simulink model "3_ALS_Sterilisation"  (R2023b)
settings: Solver=VariableStepAuto  StartTime=0.0  StopTime=312  RelTol=1e-3
libraries: fl_lib x57, nesl_utility x10, dspstat3 x1
settings Model: Creator=s01mn1  LastModifiedBy=s01mn1

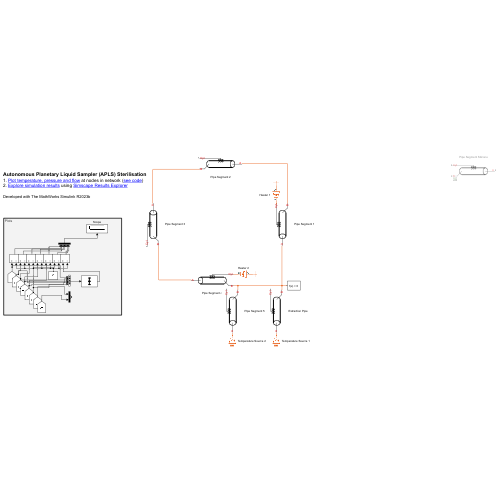
[thumbnail: Simulink's stored preview of the top-level diagram]
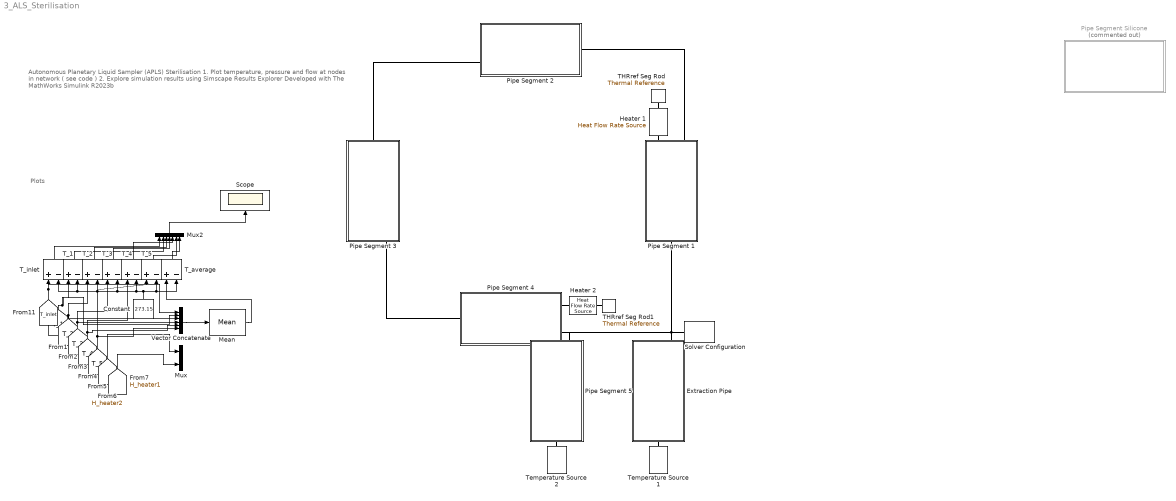
== system 3_ALS_Sterilisation ==
  note: Plots
  note: Autonomous Planetary Liquid Sampler (APLS) Sterilisation
      | 1. Plot temperature, pressure and flow at nodes in network ( see code )
      | 2. Explore simulation results using Simscape Results Explorer
      |
      | Developed with The MathWorks Simulink R2023b
  Constant : Constant  Value=273.15
  Extraction Pipe : Subsystem
      mask Display:
      | % Plot cylinder
      | plot([1,3],[1,1])
      | plot([1,3],[2,2])
      | plot(0.2*cos(0:2*pi/500:2*pi)+1,0.5*sin(0:2*pi/500:2*pi)+1.5)
      | plot(0.2*cos(-pi/2:2*pi/500:pi/2)+3,0.5*sin(-pi/2:2*pi/500:pi/2)+1.5)
      | 
      | % Heat Port
      | plot([1.8 2.2],[2.2 2.2])
      | plot([0.1*cos(-pi/2:0.1:pi/2)+1.8],[0.1*sin(-pi/2:0.1:pi/2)+2.1])
      | plot([0.1*cos(pi/2:0.1:3*pi/2)+1.9],[0.1*sin(pi/2:0.1:3*pi/2)+1.9])
      | plot([0.1*cos(-pi/2:0.1:pi/2)+1.95],[0.1*sin(-pi/2:0.1:pi/2)+2.1])
      | plot([0.1*cos(pi/2:0.1:3*pi/2)+2.05],[0.1*sin(pi/2:0.1:3*pi/2)+1.9])
      | plot([0.1*cos(-pi/2:0.1:pi/2)+2.1],[0.1*sin(-pi/2:0.1:pi/2)+2.1])
      | plot([0.1*cos(pi/2:0.1:3*pi/2)+2.2],[0.1*sin(pi/2:0.1:3*pi/2)+1.9])
      | 
      | % Connecting lines
      | plot([2 3.8],[2.4,2.4])
      | plot([2 2],[2.2 2.4])
      | plot([0.2 1],[1.5 1.5])
      | plot([3.4 3.8],[0.75 0.75])
      | plot([3,3.4],[1.5 0.75])
      | % Scaling
      | color('white')
      | plot(0.2,0)
      | plot(3.8,3.2)
      | 
      | color('red')
      | port_label('Lconn',1,'A')
      | port_label('Rconn',1,'Cyl')
      | port_label('Rconn',2,'B')
  Heater 1 : fl_lib/Thermal/Thermal Sources/Heat Flow Rate Source  heat_flow=60 W
      settings: InternalSimscapePortConfiguration="{\"Bottom\":[],\"Left\":[{\"id\":\"B\",\"label\":\"B\",\"type\":\"foundation.thermal.thermal\"}],\"Right\":[{\"id\":\"A\",\"label\":\"A\",\"type\":\"foundation.thermal.thermal\"}],\"Top\":[]}"
  Heater 2 : fl_lib/Thermal/Thermal Sources/Heat Flow Rate Source  heat_flow=60 W
      settings: InternalSimscapePortConfiguration="{\"Bottom\":[],\"Left\":[{\"id\":\"B\",\"label\":\"B\",\"type\":\"foundation.thermal.thermal\"}],\"Right\":[{\"id\":\"A\",\"label\":\"A\",\"type\":\"foundation.thermal.thermal\"}],\"Top\":[]}"
  Mean : dspstat3/Mean  run=off  InputProcessing=Columns as channels (frame based)  reset_popup=None  directionMode=Each column  dimension=1  roiEnable=off  roiType=Rectangles  roiPortion=Entire ROI  roiOutput=Individual statistics for each ROI  roiFlag=off  roundingMode=Floor  overflowMode=off  outputDataTypeStr=Inherit: Same as accumulator  outputMin=[]  outputMax=[]  outputLastDataTypeStr=Inherit: Same as accumulator
  Mux : Mux  Inputs=2
  Mux2 : Mux  Inputs=7
  Pipe Segment 1 : Subsystem
      mask Display:
      | % Plot cylinder
      | plot([1,3],[1,1])
      | plot([1,3],[2,2])
      | plot(0.2*cos(0:2*pi/500:2*pi)+1,0.5*sin(0:2*pi/500:2*pi)+1.5)
      | plot(0.2*cos(-pi/2:2*pi/500:pi/2)+3,0.5*sin(-pi/2:2*pi/500:pi/2)+1.5)
      | 
      | % Heat Port
      | plot([1.8 2.2],[2.2 2.2])
      | plot([0.1*cos(-pi/2:0.1:pi/2)+1.8],[0.1*sin(-pi/2:0.1:pi/2)+2.1])
      | plot([0.1*cos(pi/2:0.1:3*pi/2)+1.9],[0.1*sin(pi/2:0.1:3*pi/2)+1.9])
      | plot([0.1*cos(-pi/2:0.1:pi/2)+1.95],[0.1*sin(-pi/2:0.1:pi/2)+2.1])
      | plot([0.1*cos(pi/2:0.1:3*pi/2)+2.05],[0.1*sin(pi/2:0.1:3*pi/2)+1.9])
      | plot([0.1*cos(-pi/2:0.1:pi/2)+2.1],[0.1*sin(-pi/2:0.1:pi/2)+2.1])
      | plot([0.1*cos(pi/2:0.1:3*pi/2)+2.2],[0.1*sin(pi/2:0.1:3*pi/2)+1.9])
      | 
      | % Connecting lines
      | plot([2 3.8],[2.4,2.4])
      | plot([2 2],[2.2 2.4])
      | plot([0.2 1],[1.5 1.5])
      | plot([3.4 3.8],[0.75 0.75])
      | plot([3,3.4],[1.5 0.75])
      | % Scaling
      | color('white')
      | plot(0.2,0)
      | plot(3.8,3.2)
      | 
      | color('red')
      | port_label('Lconn',1,'A')
      | port_label('Rconn',1,'Cyl')
      | port_label('Rconn',2,'B')
  Pipe Segment 2 : Subsystem
      mask Display:
      | % Plot cylinder
      | plot([1,3],[1,1])
      | plot([1,3],[2,2])
      | plot(0.2*cos(0:2*pi/500:2*pi)+1,0.5*sin(0:2*pi/500:2*pi)+1.5)
      | plot(0.2*cos(-pi/2:2*pi/500:pi/2)+3,0.5*sin(-pi/2:2*pi/500:pi/2)+1.5)
      | 
      | % Heat Port
      | plot([1.8 2.2],[2.2 2.2])
      | plot([0.1*cos(-pi/2:0.1:pi/2)+1.8],[0.1*sin(-pi/2:0.1:pi/2)+2.1])
      | plot([0.1*cos(pi/2:0.1:3*pi/2)+1.9],[0.1*sin(pi/2:0.1:3*pi/2)+1.9])
      | plot([0.1*cos(-pi/2:0.1:pi/2)+1.95],[0.1*sin(-pi/2:0.1:pi/2)+2.1])
      | plot([0.1*cos(pi/2:0.1:3*pi/2)+2.05],[0.1*sin(pi/2:0.1:3*pi/2)+1.9])
      | plot([0.1*cos(-pi/2:0.1:pi/2)+2.1],[0.1*sin(-pi/2:0.1:pi/2)+2.1])
      | plot([0.1*cos(pi/2:0.1:3*pi/2)+2.2],[0.1*sin(pi/2:0.1:3*pi/2)+1.9])
      | 
      | % Connecting lines
      | plot([2 3.8],[2.4,2.4])
      | plot([2 2],[2.2 2.4])
      | plot([0.2 1],[1.5 1.5])
      | plot([3.4 3.8],[0.75 0.75])
      | plot([3,3.4],[1.5 0.75])
      | % Scaling
      | color('white')
      | plot(0.2,0)
      | plot(3.8,3.2)
      | 
      | color('red')
      | port_label('Lconn',1,'A')
      | port_label('Rconn',1,'Cyl')
      | port_label('Rconn',2,'B')
  Pipe Segment 3 : Subsystem
      mask Display:
      | % Plot cylinder
      | plot([1,3],[1,1])
      | plot([1,3],[2,2])
      | plot(0.2*cos(0:2*pi/500:2*pi)+1,0.5*sin(0:2*pi/500:2*pi)+1.5)
      | plot(0.2*cos(-pi/2:2*pi/500:pi/2)+3,0.5*sin(-pi/2:2*pi/500:pi/2)+1.5)
      | 
      | % Heat Port
      | plot([1.8 2.2],[2.2 2.2])
      | plot([0.1*cos(-pi/2:0.1:pi/2)+1.8],[0.1*sin(-pi/2:0.1:pi/2)+2.1])
      | plot([0.1*cos(pi/2:0.1:3*pi/2)+1.9],[0.1*sin(pi/2:0.1:3*pi/2)+1.9])
      | plot([0.1*cos(-pi/2:0.1:pi/2)+1.95],[0.1*sin(-pi/2:0.1:pi/2)+2.1])
      | plot([0.1*cos(pi/2:0.1:3*pi/2)+2.05],[0.1*sin(pi/2:0.1:3*pi/2)+1.9])
      | plot([0.1*cos(-pi/2:0.1:pi/2)+2.1],[0.1*sin(-pi/2:0.1:pi/2)+2.1])
      | plot([0.1*cos(pi/2:0.1:3*pi/2)+2.2],[0.1*sin(pi/2:0.1:3*pi/2)+1.9])
      | 
      | % Connecting lines
      | plot([2 3.8],[2.4,2.4])
      | plot([2 2],[2.2 2.4])
      | plot([0.2 1],[1.5 1.5])
      | plot([3.4 3.8],[0.75 0.75])
      | plot([3,3.4],[1.5 0.75])
      | % Scaling
      | color('white')
      | plot(0.2,0)
      | plot(3.8,3.2)
      | 
      | color('red')
      | port_label('Lconn',1,'A')
      | port_label('Rconn',1,'Cyl')
      | port_label('Rconn',2,'B')
  Pipe Segment 4 : Subsystem
      mask Display:
      | % Plot cylinder
      | plot([1,3],[1,1])
      | plot([1,3],[2,2])
      | plot(0.2*cos(0:2*pi/500:2*pi)+1,0.5*sin(0:2*pi/500:2*pi)+1.5)
      | plot(0.2*cos(-pi/2:2*pi/500:pi/2)+3,0.5*sin(-pi/2:2*pi/500:pi/2)+1.5)
      | 
      | % Heat Port
      | plot([1.8 2.2],[2.2 2.2])
      | plot([0.1*cos(-pi/2:0.1:pi/2)+1.8],[0.1*sin(-pi/2:0.1:pi/2)+2.1])
      | plot([0.1*cos(pi/2:0.1:3*pi/2)+1.9],[0.1*sin(pi/2:0.1:3*pi/2)+1.9])
      | plot([0.1*cos(-pi/2:0.1:pi/2)+1.95],[0.1*sin(-pi/2:0.1:pi/2)+2.1])
      | plot([0.1*cos(pi/2:0.1:3*pi/2)+2.05],[0.1*sin(pi/2:0.1:3*pi/2)+1.9])
      | plot([0.1*cos(-pi/2:0.1:pi/2)+2.1],[0.1*sin(-pi/2:0.1:pi/2)+2.1])
      | plot([0.1*cos(pi/2:0.1:3*pi/2)+2.2],[0.1*sin(pi/2:0.1:3*pi/2)+1.9])
      | 
      | % Connecting lines
      | plot([2 3.8],[2.4,2.4])
      | plot([2 2],[2.2 2.4])
      | plot([0.2 1],[1.5 1.5])
      | plot([3.4 3.8],[0.75 0.75])
      | plot([3,3.4],[1.5 0.75])
      | % Scaling
      | color('white')
      | plot(0.2,0)
      | plot(3.8,3.2)
      | 
      | color('red')
      | port_label('Lconn',1,'A')
      | port_label('Rconn',1,'Cyl')
      | port_label('Rconn',2,'B')
  Pipe Segment 5 : Subsystem
      mask Display:
      | % Plot cylinder
      | plot([1,3],[1,1])
      | plot([1,3],[2,2])
      | plot(0.2*cos(0:2*pi/500:2*pi)+1,0.5*sin(0:2*pi/500:2*pi)+1.5)
      | plot(0.2*cos(-pi/2:2*pi/500:pi/2)+3,0.5*sin(-pi/2:2*pi/500:pi/2)+1.5)
      | 
      | % Heat Port
      | plot([1.8 2.2],[2.2 2.2])
      | plot([0.1*cos(-pi/2:0.1:pi/2)+1.8],[0.1*sin(-pi/2:0.1:pi/2)+2.1])
      | plot([0.1*cos(pi/2:0.1:3*pi/2)+1.9],[0.1*sin(pi/2:0.1:3*pi/2)+1.9])
      | plot([0.1*cos(-pi/2:0.1:pi/2)+1.95],[0.1*sin(-pi/2:0.1:pi/2)+2.1])
      | plot([0.1*cos(pi/2:0.1:3*pi/2)+2.05],[0.1*sin(pi/2:0.1:3*pi/2)+1.9])
      | plot([0.1*cos(-pi/2:0.1:pi/2)+2.1],[0.1*sin(-pi/2:0.1:pi/2)+2.1])
      | plot([0.1*cos(pi/2:0.1:3*pi/2)+2.2],[0.1*sin(pi/2:0.1:3*pi/2)+1.9])
      | 
      | % Connecting lines
      | plot([2 3.8],[2.4,2.4])
      | plot([2 2],[2.2 2.4])
      | plot([0.2 1],[1.5 1.5])
      | plot([3.4 3.8],[0.75 0.75])
      | plot([3,3.4],[1.5 0.75])
      | % Scaling
      | color('white')
      | plot(0.2,0)
      | plot(3.8,3.2)
      | 
      | color('red')
      | port_label('Lconn',1,'A')
      | port_label('Rconn',1,'Cyl')
      | port_label('Rconn',2,'B')
  Pipe Segment Silicone : Subsystem  Commented=on
      mask Display:
      | % Plot cylinder
      | plot([1,3],[1,1])
      | plot([1,3],[2,2])
      | plot(0.2*cos(0:2*pi/500:2*pi)+1,0.5*sin(0:2*pi/500:2*pi)+1.5)
      | plot(0.2*cos(-pi/2:2*pi/500:pi/2)+3,0.5*sin(-pi/2:2*pi/500:pi/2)+1.5)
      | 
      | % Heat Port
      | plot([1.8 2.2],[2.2 2.2])
      | plot([0.1*cos(-pi/2:0.1:pi/2)+1.8],[0.1*sin(-pi/2:0.1:pi/2)+2.1])
      | plot([0.1*cos(pi/2:0.1:3*pi/2)+1.9],[0.1*sin(pi/2:0.1:3*pi/2)+1.9])
      | plot([0.1*cos(-pi/2:0.1:pi/2)+1.95],[0.1*sin(-pi/2:0.1:pi/2)+2.1])
      | plot([0.1*cos(pi/2:0.1:3*pi/2)+2.05],[0.1*sin(pi/2:0.1:3*pi/2)+1.9])
      | plot([0.1*cos(-pi/2:0.1:pi/2)+2.1],[0.1*sin(-pi/2:0.1:pi/2)+2.1])
      | plot([0.1*cos(pi/2:0.1:3*pi/2)+2.2],[0.1*sin(pi/2:0.1:3*pi/2)+1.9])
      | 
      | % Connecting lines
      | plot([2 3.8],[2.4,2.4])
      | plot([2 2],[2.2 2.4])
      | plot([0.2 1],[1.5 1.5])
      | plot([3.4 3.8],[0.75 0.75])
      | plot([3,3.4],[1.5 0.75])
      | % Scaling
      | color('white')
      | plot(0.2,0)
      | plot(3.8,3.2)
      | 
      | color('red')
      | port_label('Lconn',1,'A')
      | port_label('Rconn',1,'Cyl')
      | port_label('Rconn',2,'B')
  Scope : Scope
  Solver Configuration : nesl_utility/Solver Configuration  PhysicalDomain=network_engine_domain  SubClassName=solver  LeftPortType=input  RightPortType=generic  Tones=[]  Harmonics=[]  SimulateNoise=off  Profile=off  UseLocalSampling=off  EnableSwitchedLinearOptims=on  FrequencyDomain=off  UseCCode=off  RelTol=0.001  AbsTol=0.001  MinStep=1e-09  ToWorkspace=off  RevertToSquareIcSolve=off  NumHomotopyIterations=100  PhasorMode=off  PhasorModeNumHarmonics=1  ConsistencySolver=NEWTON_XTOL_AFTER_FTOL  IndexReductionMethod=DerivativeReplacement  DoDC=off  ResidualTolerance=1e-09  ConsistencyTolSource=GLOBAL  ConsistencyAbsTol=0.001  ConsistencyRelTol=0.001  ConsistencyTolFactor=0.001  UseLocalSolver=off  LocalSolverChoice=NE_BACKWARD_EULER_ADVANCER  ResolveIndetEquations=on  FunctionEvalNumThread=1  LocalSolverSampleTime=0.001  DoFixedCost=off  MaxNonlinIter=3  MaxModeIter=2  ComputeImpulses=off  ImpulseIterations=2  LinearAlgebra=auto  LinearAlgebraNumThread=0  EquationFormulation=NE_TIME_EF  DelaysMemoryBudget=1024  AutomaticFiltering=on  FilteringTimeConstant=0.001  PartitionStorageMethod=AS_NEEDED  PartitionMemoryBudget=1024  PartitionMethod=ROBUST  MultibodyUseLocalSolver=off  MultibodyLocalSolverChoice=ODE1  MultibodyLocalSolverSampleTime=0.001
  THRref Seg Rod : fl_lib/Thermal/Thermal Elements/Thermal Reference
  THRref Seg Rod1 : fl_lib/Thermal/Thermal Elements/Thermal Reference
  T_{1..5} (5 alike) : Sum  Inputs=+-
  T_average : Sum  Inputs=+-
  T_inlet : Sum  Inputs=+-
  Temperature Source 1 : fl_lib/Thermal/Thermal Sources/Temperature Source  temperature=30 degC
  Temperature Source 2 : fl_lib/Thermal/Thermal Sources/Temperature Source  temperature=30 degC
  Vector Concatenate : Concatenate  NumInputs=6
  wires:
  Constant/1 -> T_inlet/2, T_1/2, T_2/2, T_3/2, T_4/2, T_average/2, T_5/2
  Mux2/1 -> Scope/1
  [T_inlet] -> Vector Concatenate/1, T_inlet/1
  [T_1] -> Vector Concatenate/2, T_1/1
  [T_2] -> T_2/1, Vector Concatenate/3
  [T_3] -> T_3/1, Vector Concatenate/4
  T_inlet/1 -> Mux2/1
  T_1/1 -> Mux2/2
  T_2/1 -> Mux2/3
  T_3/1 -> Mux2/4
  [T_4] -> Vector Concatenate/5, T_4/1
  T_4/1 -> Mux2/5
  [T_5] -> Vector Concatenate/6, T_5/1
  T_5/1 -> Mux2/6
  [H_heater2] -> Mux/1
  [H_heater1] -> Mux/2
  T_average/1 -> Mux2/7
  Vector Concatenate/1 -> Mean/1
  Mean/1 -> T_average/1
  connections:
  Heater 1/LConn1 -- Pipe Segment 1/RConn1
  THRref Seg Rod/LConn1 -- Heater 1/RConn1
  Solver Configuration/RConn1 -- Pipe Segment 4/RConn2 -- Pipe Segment 5/RConn2 -- Extraction Pipe/RConn2 -- Pipe Segment 1/LConn1
  Pipe Segment 4/LConn1 -- Pipe Segment 3/RConn2
  THRref Seg Rod1/LConn1 -- Heater 2/RConn1
  Heater 2/LConn1 -- Pipe Segment 4/RConn1
  Pipe Segment 3/LConn1 -- Pipe Segment 2/RConn2
  Pipe Segment 2/LConn1 -- Pipe Segment 1/RConn2
  Temperature Source 1/LConn1 -- Extraction Pipe/LConn1
  Temperature Source 2/LConn1 -- Pipe Segment 5/LConn1

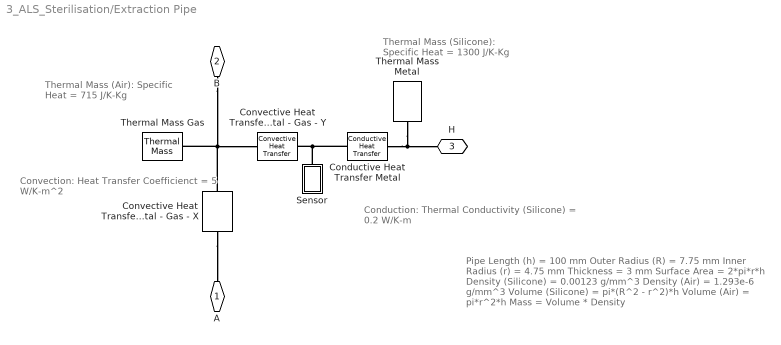
== system 3_ALS_Sterilisation/Extraction Pipe ==
  note: Thermal Mass (Silicone):
      | Specific Heat = 1300 J/K-Kg
  note: Thermal Mass  (Air):
      | Specific Heat = 715 J/K-Kg
  note: Pipe Length (h) = 100 mm
      | Outer Radius (R) = 7.75 mm
      | Inner Radius (r) = 4.75 mm
      | Thickness = 3 mm
      | Surface Area = 2*pi*r*h
      | Density (Silicone) = 0.00123 g/mm^3
      | Density (Air) = 1.293e-6 g/mm^3
      | Volume (Silicone) = pi*(R^2 - r^2)*h
      | Volume (Air) = pi*r^2*h
      | Mass = Volume * Density
  note: Conduction:
      | Thermal Conductivity (Silicone) = 0.2 W/K-m
  note: Convection:
      | Heat Transfer Coefficienct = 5 W/K-m^2
  Conductive Heat Transfer Metal : fl_lib/Thermal/Thermal Elements/Conductive Heat Transfer  thermal_type=foundation.enum.ConstantVariableTabulated.Constant  wall_geometry=foundation.enum.ConductionWallGeometry.Planar  area=7461.282 mm^2  thickness=3 mm  d_in=0.05 m  d_out=0.1 m  L=1 m  th_cond_min=10 W/(K*m)  th_cond=0.2 W/(K*m)  th_cond_TLU=[413, 401, 392, 383, 371, 357, 342] W/(K*m)  temp_TLU=[200, 273, 400, 600, 800, 1000, 1200] K  T_specify=on  T_priority=None  T=30 degC  T_nominal_specify=off  T_nominal_unit=K  T_nominal_value=1  Q_specify=off  Q_priority=None  Q=0 W  Q_nominal_specify=off  Q_nominal_unit=W  Q_nominal_value=1
  Convective Heat Transfer Metal - Gas - X : fl_lib/Thermal/Thermal Elements/Convective Heat Transfer  thermal_type=foundation.enum.constant_variable.constant  area=7461.282 mm^2  heat_tr_coeff=5 W/(K*m^2)  min_heat_tr_coeff=1e-3 W/(K*m^2)  T_specify=on  T_priority=None  T=30 degC  T_nominal_specify=off  T_nominal_unit=K  T_nominal_value=1  Q_specify=off  Q_priority=None  Q=0 W  Q_nominal_specify=off  Q_nominal_unit=W  Q_nominal_value=1
  Convective Heat Transfer Metal - Gas - Y : fl_lib/Thermal/Thermal Elements/Convective Heat Transfer  thermal_type=foundation.enum.constant_variable.constant  area=7461.282 mm^2  heat_tr_coeff=5 W/(K*m^2)  min_heat_tr_coeff=1e-3 W/(K*m^2)  T_specify=on  T_priority=None  T=30 degC  T_nominal_specify=off  T_nominal_unit=K  T_nominal_value=1  Q_specify=off  Q_priority=None  Q=0 W  Q_nominal_specify=off  Q_nominal_unit=W  Q_nominal_value=1
  Sensor : Subsystem
  Thermal Mass Gas : fl_lib/Thermal/Thermal Elements/Thermal Mass  mass_type=foundation.enum.constant_variable.constant  mass=0.0229 g  sp_heat=715 J/(K*kg)  mass_min=1e-6 kg  num_ports=foundation.enum.numPorts2.one  m_specify=off  m_priority=High  m=1 kg  m_nominal_specify=off  m_nominal_unit=kg  m_nominal_value=1  T_specify=on  T_priority=High  T=30 degC  T_nominal_specify=off  T_nominal_unit=K  T_nominal_value=1  Q_specify=off  Q_priority=None  Q=0 W  Q_nominal_specify=off  Q_nominal_unit=W  Q_nominal_value=1
  Thermal Mass Metal : fl_lib/Thermal/Thermal Elements/Thermal Mass  mass_type=foundation.enum.constant_variable.constant  mass=36.2265 g  sp_heat=1300 J/(K*kg)  mass_min=1e-6 kg  num_ports=foundation.enum.numPorts2.one  m_specify=off  m_priority=High  m=1 kg  m_nominal_specify=off  m_nominal_unit=kg  m_nominal_value=1  T_specify=on  T_priority=High  T=30 degC  T_nominal_specify=off  T_nominal_unit=K  T_nominal_value=1  Q_specify=off  Q_priority=None  Q=0 W  Q_nominal_specify=off  Q_nominal_unit=W  Q_nominal_value=1
  A : PMIOPort  Side=Left
  B : PMIOPort  Port=2  Side=Right
  H : PMIOPort  Port=3  Side=Right
  connections:
  Thermal Mass Metal/LConn1 -- H/RConn1 -- Conductive Heat Transfer Metal/LConn1
  Convective Heat Transfer Metal - Gas - X/RConn1 -- Thermal Mass Gas/LConn1 -- Convective Heat Transfer Metal - Gas - Y/RConn1 -- B/RConn1
  Sensor/LConn1 -- Convective Heat Transfer Metal - Gas - Y/LConn1 -- Conductive Heat Transfer Metal/RConn1
  Convective Heat Transfer Metal - Gas - X/LConn1 -- A/RConn1

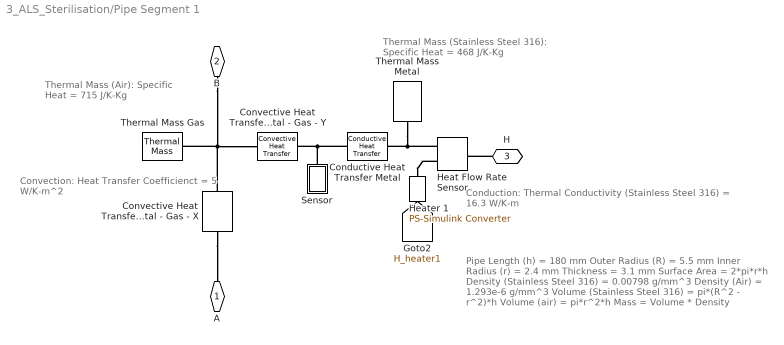
== system 3_ALS_Sterilisation/Pipe Segment 1 ==
  note: Pipe Length (h) = 180 mm
      | Outer Radius (R) = 5.5 mm
      | Inner Radius (r) = 2.4 mm
      | Thickness = 3.1 mm
      | Surface Area = 2*pi*r*h
      | Density (Stainless Steel 316) = 0.00798 g/mm^3
      | Density (Air) = 1.293e-6 g/mm^3
      | Volume (Stainless Steel 316) = pi*(R^2 - r^2)*h
      | Volume (air) = pi*r^2*h
      | Mass = Volume * Density
  note: Thermal Mass (Stainless Steel 316):
      | Specific Heat = 468 J/K-Kg
  note: Conduction:
      | Thermal Conductivity (Stainless Steel 316) = 16.3 W/K-m
  note: Convection:
      | Heat Transfer Coefficienct = 5 W/K-m^2
  note: Thermal Mass  (Air):
      | Specific Heat = 715 J/K-Kg
  Conductive Heat Transfer Metal : fl_lib/Thermal/Thermal Elements/Conductive Heat Transfer  thermal_type=foundation.enum.ConstantVariableTabulated.Constant  wall_geometry=foundation.enum.ConductionWallGeometry.Planar  area=2714.336 mm^2  thickness=3.1 mm  d_in=0.05 m  d_out=0.1 m  L=1 m  th_cond_min=10 W/(K*m)  th_cond=16.3 W/(K*m)  th_cond_TLU=[413, 401, 392, 383, 371, 357, 342] W/(K*m)  temp_TLU=[200, 273, 400, 600, 800, 1000, 1200] K  T_specify=on  T_priority=None  T=30 degC  T_nominal_specify=off  T_nominal_unit=K  T_nominal_value=1  Q_specify=off  Q_priority=None  Q=0 W  Q_nominal_specify=off  Q_nominal_unit=W  Q_nominal_value=1
  Convective Heat Transfer Metal - Gas - X : fl_lib/Thermal/Thermal Elements/Convective Heat Transfer  thermal_type=foundation.enum.constant_variable.constant  area=2714.336 mm^2  heat_tr_coeff=5 W/(K*m^2)  min_heat_tr_coeff=1e-3 W/(K*m^2)  T_specify=on  T_priority=None  T=30 degC  T_nominal_specify=off  T_nominal_unit=K  T_nominal_value=1  Q_specify=off  Q_priority=None  Q=0 W  Q_nominal_specify=off  Q_nominal_unit=W  Q_nominal_value=1
  Convective Heat Transfer Metal - Gas - Y : fl_lib/Thermal/Thermal Elements/Convective Heat Transfer  thermal_type=foundation.enum.constant_variable.constant  area=2714.336 mm^2  heat_tr_coeff=5 W/(K*m^2)  min_heat_tr_coeff=1e-3 W/(K*m^2)  T_specify=on  T_priority=None  T=30 degC  T_nominal_specify=off  T_nominal_unit=K  T_nominal_value=1  Q_specify=off  Q_priority=None  Q=0 W  Q_nominal_specify=off  Q_nominal_unit=W  Q_nominal_value=1
  Heat Flow Rate Sensor : fl_lib/Thermal/Thermal Sensors/Heat Flow Rate Sensor
  Heater 1 : nesl_utility/PS-Simulink Converter  PhysicalDomain=network_engine_domain  SubClassName=ps_output  LeftPortType=input  RightPortType=output  PseudoPeriodic=off  Frequencies=[]  VectorFormat=inherit  Unit=inherit  AffineConversion=off
  Sensor : Subsystem
  Thermal Mass Gas : fl_lib/Thermal/Thermal Elements/Thermal Mass  mass_type=foundation.enum.constant_variable.constant  mass=0.0042 g  sp_heat=715 J/(K*kg)  mass_min=1e-6 kg  num_ports=foundation.enum.numPorts2.one  m_specify=off  m_priority=High  m=1 kg  m_nominal_specify=off  m_nominal_unit=kg  m_nominal_value=1  T_specify=on  T_priority=High  T=30 degC  T_nominal_specify=off  T_nominal_unit=K  T_nominal_value=1  Q_specify=off  Q_priority=None  Q=0 W  Q_nominal_specify=off  Q_nominal_unit=W  Q_nominal_value=1
  Thermal Mass Metal : fl_lib/Thermal/Thermal Elements/Thermal Mass  mass_type=foundation.enum.constant_variable.constant  mass=110.5132 g  sp_heat=468 J/(K*kg)  mass_min=1e-6 kg  num_ports=foundation.enum.numPorts2.one  m_specify=off  m_priority=High  m=1 kg  m_nominal_specify=off  m_nominal_unit=kg  m_nominal_value=1  T_specify=on  T_priority=High  T=30 degC  T_nominal_specify=off  T_nominal_unit=K  T_nominal_value=1  Q_specify=off  Q_priority=None  Q=0 W  Q_nominal_specify=off  Q_nominal_unit=W  Q_nominal_value=1
  A : PMIOPort  Side=Left
  B : PMIOPort  Port=2  Side=Right
  H : PMIOPort  Port=3  Side=Right
  tag scope: H_heater1=global
  wires:
  Heater 1/1 -> [H_heater1]
  connections:
  Conductive Heat Transfer Metal/RConn1 -- Convective Heat Transfer Metal - Gas - Y/LConn1 -- Sensor/LConn1
  Thermal Mass Metal/LConn1 -- Heat Flow Rate Sensor/RConn2 -- Conductive Heat Transfer Metal/LConn1
  Convective Heat Transfer Metal - Gas - X/LConn1 -- A/RConn1
  Convective Heat Transfer Metal - Gas - X/RConn1 -- B/RConn1 -- Thermal Mass Gas/LConn1 -- Convective Heat Transfer Metal - Gas - Y/RConn1
  Heat Flow Rate Sensor/RConn1 -- Heater 1/LConn1
  H/RConn1 -- Heat Flow Rate Sensor/LConn1

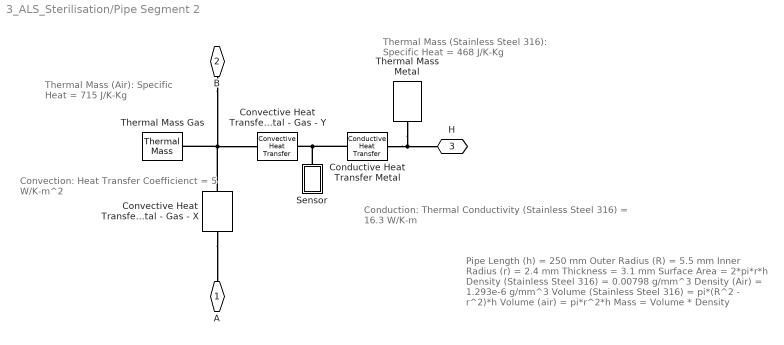
== system 3_ALS_Sterilisation/Pipe Segment 2 ==
  note: Convection:
      | Heat Transfer Coefficienct = 5 W/K-m^2
  note: Thermal Mass (Stainless Steel 316):
      | Specific Heat = 468 J/K-Kg
  note: Conduction:
      | Thermal Conductivity (Stainless Steel 316) = 16.3 W/K-m
  note: Thermal Mass  (Air):
      | Specific Heat = 715 J/K-Kg
  note: Pipe Length (h) = 250 mm
      | Outer Radius (R) = 5.5 mm
      | Inner Radius (r) = 2.4 mm
      | Thickness = 3.1 mm
      | Surface Area = 2*pi*r*h
      | Density (Stainless Steel 316) = 0.00798 g/mm^3
      | Density (Air) = 1.293e-6 g/mm^3
      | Volume (Stainless Steel 316) = pi*(R^2 - r^2)*h
      | Volume (air) = pi*r^2*h
      | Mass = Volume * Density
  Conductive Heat Transfer Metal : fl_lib/Thermal/Thermal Elements/Conductive Heat Transfer  thermal_type=foundation.enum.ConstantVariableTabulated.Constant  wall_geometry=foundation.enum.ConductionWallGeometry.Planar  area=3769.911 mm^2  thickness=3.1 mm  d_in=0.05 m  d_out=0.1 m  L=1 m  th_cond_min=10 W/(K*m)  th_cond=16.3 W/(K*m)  th_cond_TLU=[413, 401, 392, 383, 371, 357, 342] W/(K*m)  temp_TLU=[200, 273, 400, 600, 800, 1000, 1200] K  T_specify=on  T_priority=None  T=30 degC  T_nominal_specify=off  T_nominal_unit=K  T_nominal_value=1  Q_specify=off  Q_priority=None  Q=0 W  Q_nominal_specify=off  Q_nominal_unit=W  Q_nominal_value=1
  Convective Heat Transfer Metal - Gas - X : fl_lib/Thermal/Thermal Elements/Convective Heat Transfer  thermal_type=foundation.enum.constant_variable.constant  area=3769.911 mm^2  heat_tr_coeff=5 W/(K*m^2)  min_heat_tr_coeff=1e-3 W/(K*m^2)  T_specify=on  T_priority=None  T=30 degC  T_nominal_specify=off  T_nominal_unit=K  T_nominal_value=1  Q_specify=off  Q_priority=None  Q=0 W  Q_nominal_specify=off  Q_nominal_unit=W  Q_nominal_value=1
  Convective Heat Transfer Metal - Gas - Y : fl_lib/Thermal/Thermal Elements/Convective Heat Transfer  thermal_type=foundation.enum.constant_variable.constant  area=3769.911 mm^2  heat_tr_coeff=5 W/(K*m^2)  min_heat_tr_coeff=1e-3 W/(K*m^2)  T_specify=on  T_priority=None  T=30 degC  T_nominal_specify=off  T_nominal_unit=K  T_nominal_value=1  Q_specify=off  Q_priority=None  Q=0 W  Q_nominal_specify=off  Q_nominal_unit=W  Q_nominal_value=1
  Sensor : Subsystem
  Thermal Mass Gas : fl_lib/Thermal/Thermal Elements/Thermal Mass  mass_type=foundation.enum.constant_variable.constant  mass=0.0058 g  sp_heat=715 J/(K*kg)  mass_min=1e-6 kg  num_ports=foundation.enum.numPorts2.one  m_specify=off  m_priority=High  m=1 kg  m_nominal_specify=off  m_nominal_unit=kg  m_nominal_value=1  T_specify=on  T_priority=High  T=30 degC  T_nominal_specify=off  T_nominal_unit=K  T_nominal_value=1  Q_specify=off  Q_priority=None  Q=0 W  Q_nominal_specify=off  Q_nominal_unit=W  Q_nominal_value=1
  Thermal Mass Metal : fl_lib/Thermal/Thermal Elements/Thermal Mass  mass_type=foundation.enum.constant_variable.constant  mass=153.4905 g  sp_heat=468 J/(K*kg)  mass_min=1e-6 kg  num_ports=foundation.enum.numPorts2.one  m_specify=off  m_priority=High  m=1 kg  m_nominal_specify=off  m_nominal_unit=kg  m_nominal_value=1  T_specify=on  T_priority=High  T=30 degC  T_nominal_specify=off  T_nominal_unit=K  T_nominal_value=1  Q_specify=off  Q_priority=None  Q=0 W  Q_nominal_specify=off  Q_nominal_unit=W  Q_nominal_value=1
  A : PMIOPort  Side=Left
  B : PMIOPort  Port=2  Side=Right
  H : PMIOPort  Port=3  Side=Right
  connections:
  Convective Heat Transfer Metal - Gas - X/RConn1 -- Thermal Mass Gas/LConn1 -- Convective Heat Transfer Metal - Gas - Y/RConn1 -- B/RConn1
  Sensor/LConn1 -- Convective Heat Transfer Metal - Gas - Y/LConn1 -- Conductive Heat Transfer Metal/RConn1
  Thermal Mass Metal/LConn1 -- H/RConn1 -- Conductive Heat Transfer Metal/LConn1
  Convective Heat Transfer Metal - Gas - X/LConn1 -- A/RConn1

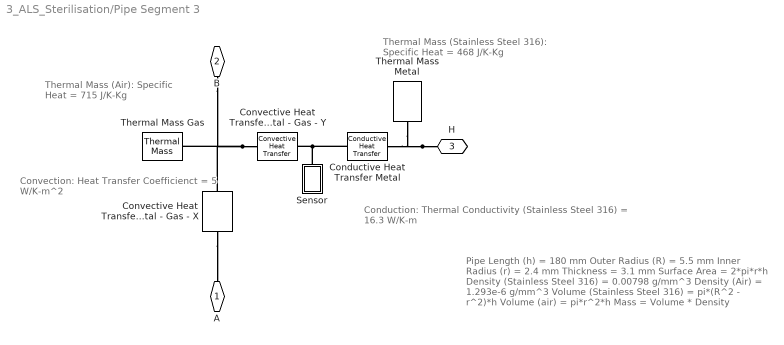
== system 3_ALS_Sterilisation/Pipe Segment 3 ==
  note: Thermal Mass (Stainless Steel 316):
      | Specific Heat = 468 J/K-Kg
  note: Thermal Mass  (Air):
      | Specific Heat = 715 J/K-Kg
  note: Pipe Length (h) = 180 mm
      | Outer Radius (R) = 5.5 mm
      | Inner Radius (r) = 2.4 mm
      | Thickness = 3.1 mm
      | Surface Area = 2*pi*r*h
      | Density (Stainless Steel 316) = 0.00798 g/mm^3
      | Density (Air) = 1.293e-6 g/mm^3
      | Volume (Stainless Steel 316) = pi*(R^2 - r^2)*h
      | Volume (air) = pi*r^2*h
      | Mass = Volume * Density
  note: Conduction:
      | Thermal Conductivity (Stainless Steel 316) = 16.3 W/K-m
  note: Convection:
      | Heat Transfer Coefficienct = 5 W/K-m^2
  Conductive Heat Transfer Metal : fl_lib/Thermal/Thermal Elements/Conductive Heat Transfer  thermal_type=foundation.enum.ConstantVariableTabulated.Constant  wall_geometry=foundation.enum.ConductionWallGeometry.Planar  area=2714.336 mm^2  thickness=3.1 mm  d_in=0.05 m  d_out=0.1 m  L=1 m  th_cond_min=10 W/(K*m)  th_cond=16.3 W/(K*m)  th_cond_TLU=[413, 401, 392, 383, 371, 357, 342] W/(K*m)  temp_TLU=[200, 273, 400, 600, 800, 1000, 1200] K  T_specify=on  T_priority=None  T=30 degC  T_nominal_specify=off  T_nominal_unit=K  T_nominal_value=1  Q_specify=off  Q_priority=None  Q=0 W  Q_nominal_specify=off  Q_nominal_unit=W  Q_nominal_value=1
  Convective Heat Transfer Metal - Gas - X : fl_lib/Thermal/Thermal Elements/Convective Heat Transfer  thermal_type=foundation.enum.constant_variable.constant  area=2714.336 mm^2  heat_tr_coeff=5 W/(K*m^2)  min_heat_tr_coeff=1e-3 W/(K*m^2)  T_specify=on  T_priority=None  T=30 degC  T_nominal_specify=off  T_nominal_unit=K  T_nominal_value=1  Q_specify=off  Q_priority=None  Q=0 W  Q_nominal_specify=off  Q_nominal_unit=W  Q_nominal_value=1
  Convective Heat Transfer Metal - Gas - Y : fl_lib/Thermal/Thermal Elements/Convective Heat Transfer  thermal_type=foundation.enum.constant_variable.constant  area=2714.336 mm^2  heat_tr_coeff=5 W/(K*m^2)  min_heat_tr_coeff=1e-3 W/(K*m^2)  T_specify=on  T_priority=None  T=30 degC  T_nominal_specify=off  T_nominal_unit=K  T_nominal_value=1  Q_specify=off  Q_priority=None  Q=0 W  Q_nominal_specify=off  Q_nominal_unit=W  Q_nominal_value=1
  Sensor : Subsystem
  Thermal Mass Gas : fl_lib/Thermal/Thermal Elements/Thermal Mass  mass_type=foundation.enum.constant_variable.constant  mass=0.0042 g  sp_heat=715 J/(K*kg)  mass_min=1e-6 kg  num_ports=foundation.enum.numPorts2.one  m_specify=off  m_priority=High  m=1 kg  m_nominal_specify=off  m_nominal_unit=kg  m_nominal_value=1  T_specify=on  T_priority=High  T=30 degC  T_nominal_specify=off  T_nominal_unit=K  T_nominal_value=1  Q_specify=off  Q_priority=None  Q=0 W  Q_nominal_specify=off  Q_nominal_unit=W  Q_nominal_value=1
  Thermal Mass Metal : fl_lib/Thermal/Thermal Elements/Thermal Mass  mass_type=foundation.enum.constant_variable.constant  mass=110.5132 g  sp_heat=468 J/(K*kg)  mass_min=1e-6 kg  num_ports=foundation.enum.numPorts2.one  m_specify=off  m_priority=High  m=1 kg  m_nominal_specify=off  m_nominal_unit=kg  m_nominal_value=1  T_specify=on  T_priority=High  T=30 degC  T_nominal_specify=off  T_nominal_unit=K  T_nominal_value=1  Q_specify=off  Q_priority=None  Q=0 W  Q_nominal_specify=off  Q_nominal_unit=W  Q_nominal_value=1
  A : PMIOPort  Side=Left
  B : PMIOPort  Port=2  Side=Right
  H : PMIOPort  Port=3  Side=Right
  connections:
  H/RConn1 -- Conductive Heat Transfer Metal/LConn1 -- Thermal Mass Metal/LConn1
  Convective Heat Transfer Metal - Gas - Y/RConn1 -- B/RConn1 -- Convective Heat Transfer Metal - Gas - X/RConn1 -- Thermal Mass Gas/LConn1
  Convective Heat Transfer Metal - Gas - Y/LConn1 -- Conductive Heat Transfer Metal/RConn1 -- Sensor/LConn1
  Convective Heat Transfer Metal - Gas - X/LConn1 -- A/RConn1

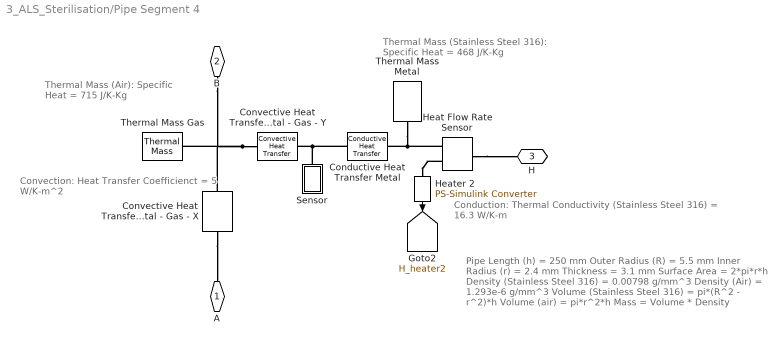
== system 3_ALS_Sterilisation/Pipe Segment 4 ==
  note: Convection:
      | Heat Transfer Coefficienct = 5 W/K-m^2
  note: Thermal Mass (Stainless Steel 316):
      | Specific Heat = 468 J/K-Kg
  note: Conduction:
      | Thermal Conductivity (Stainless Steel 316) = 16.3 W/K-m
  note: Thermal Mass  (Air):
      | Specific Heat = 715 J/K-Kg
  note: Pipe Length (h) = 250 mm
      | Outer Radius (R) = 5.5 mm
      | Inner Radius (r) = 2.4 mm
      | Thickness = 3.1 mm
      | Surface Area = 2*pi*r*h
      | Density (Stainless Steel 316) = 0.00798 g/mm^3
      | Density (Air) = 1.293e-6 g/mm^3
      | Volume (Stainless Steel 316) = pi*(R^2 - r^2)*h
      | Volume (air) = pi*r^2*h
      | Mass = Volume * Density
  Conductive Heat Transfer Metal : fl_lib/Thermal/Thermal Elements/Conductive Heat Transfer  thermal_type=foundation.enum.ConstantVariableTabulated.Constant  wall_geometry=foundation.enum.ConductionWallGeometry.Planar  area=3769.911 mm^2  thickness=3.1 mm  d_in=0.05 m  d_out=0.1 m  L=1 m  th_cond_min=10 W/(K*m)  th_cond=16.3 W/(K*m)  th_cond_TLU=[413, 401, 392, 383, 371, 357, 342] W/(K*m)  temp_TLU=[200, 273, 400, 600, 800, 1000, 1200] K  T_specify=on  T_priority=None  T=30 degC  T_nominal_specify=off  T_nominal_unit=K  T_nominal_value=1  Q_specify=off  Q_priority=None  Q=0 W  Q_nominal_specify=off  Q_nominal_unit=W  Q_nominal_value=1
  Convective Heat Transfer Metal - Gas - X : fl_lib/Thermal/Thermal Elements/Convective Heat Transfer  thermal_type=foundation.enum.constant_variable.constant  area=3769.911 mm^2  heat_tr_coeff=5 W/(K*m^2)  min_heat_tr_coeff=1e-3 W/(K*m^2)  T_specify=on  T_priority=None  T=30 degC  T_nominal_specify=off  T_nominal_unit=K  T_nominal_value=1  Q_specify=off  Q_priority=None  Q=0 W  Q_nominal_specify=off  Q_nominal_unit=W  Q_nominal_value=1
  Convective Heat Transfer Metal - Gas - Y : fl_lib/Thermal/Thermal Elements/Convective Heat Transfer  thermal_type=foundation.enum.constant_variable.constant  area=3769.911 mm^2  heat_tr_coeff=5 W/(K*m^2)  min_heat_tr_coeff=1e-3 W/(K*m^2)  T_specify=on  T_priority=None  T=30 degC  T_nominal_specify=off  T_nominal_unit=K  T_nominal_value=1  Q_specify=off  Q_priority=None  Q=0 W  Q_nominal_specify=off  Q_nominal_unit=W  Q_nominal_value=1
  Heat Flow Rate Sensor : fl_lib/Thermal/Thermal Sensors/Heat Flow Rate Sensor
  Heater 2 : nesl_utility/PS-Simulink Converter  PhysicalDomain=network_engine_domain  SubClassName=ps_output  LeftPortType=input  RightPortType=output  PseudoPeriodic=off  Frequencies=[]  VectorFormat=inherit  Unit=inherit  AffineConversion=off
  Sensor : Subsystem
  Thermal Mass Gas : fl_lib/Thermal/Thermal Elements/Thermal Mass  mass_type=foundation.enum.constant_variable.constant  mass=0.0058 g  sp_heat=715 J/(K*kg)  mass_min=1e-6 kg  num_ports=foundation.enum.numPorts2.one  m_specify=off  m_priority=High  m=1 kg  m_nominal_specify=off  m_nominal_unit=kg  m_nominal_value=1  T_specify=on  T_priority=High  T=20 degC  T_nominal_specify=off  T_nominal_unit=K  T_nominal_value=1  Q_specify=off  Q_priority=None  Q=0 W  Q_nominal_specify=off  Q_nominal_unit=W  Q_nominal_value=1
  Thermal Mass Metal : fl_lib/Thermal/Thermal Elements/Thermal Mass  mass_type=foundation.enum.constant_variable.constant  mass=153.4905 g  sp_heat=468 J/(K*kg)  mass_min=1e-6 kg  num_ports=foundation.enum.numPorts2.one  m_specify=off  m_priority=High  m=1 kg  m_nominal_specify=off  m_nominal_unit=kg  m_nominal_value=1  T_specify=on  T_priority=High  T=20 degC  T_nominal_specify=off  T_nominal_unit=K  T_nominal_value=1  Q_specify=off  Q_priority=None  Q=0 W  Q_nominal_specify=off  Q_nominal_unit=W  Q_nominal_value=1
  A : PMIOPort  Side=Left
  B : PMIOPort  Port=2  Side=Right
  H : PMIOPort  Port=3  Side=Right
  tag scope: H_heater2=global
  wires:
  Heater 2/1 -> [H_heater2]
  connections:
  Convective Heat Transfer Metal - Gas - Y/RConn1 -- B/RConn1 -- Convective Heat Transfer Metal - Gas - X/RConn1 -- Thermal Mass Gas/LConn1
  Convective Heat Transfer Metal - Gas - Y/LConn1 -- Conductive Heat Transfer Metal/RConn1 -- Sensor/LConn1
  Thermal Mass Metal/LConn1 -- Conductive Heat Transfer Metal/LConn1 -- Heat Flow Rate Sensor/RConn2
  Convective Heat Transfer Metal - Gas - X/LConn1 -- A/RConn1
  Heat Flow Rate Sensor/RConn1 -- Heater 2/LConn1
  Heat Flow Rate Sensor/LConn1 -- H/RConn1

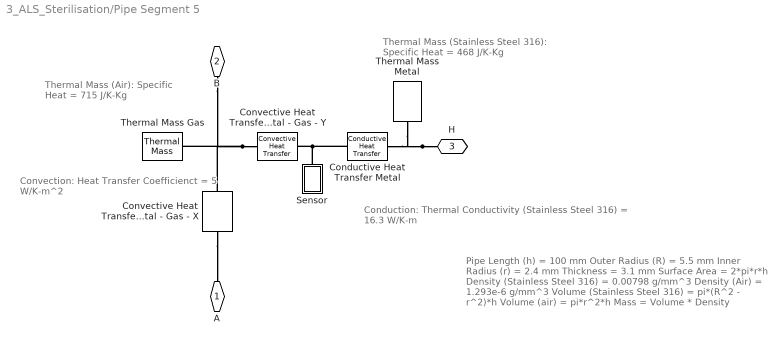
== system 3_ALS_Sterilisation/Pipe Segment 5 ==
  note: Thermal Mass (Stainless Steel 316):
      | Specific Heat = 468 J/K-Kg
  note: Thermal Mass  (Air):
      | Specific Heat = 715 J/K-Kg
  note: Pipe Length (h) = 100 mm
      | Outer Radius (R) = 5.5 mm
      | Inner Radius (r) = 2.4 mm
      | Thickness = 3.1 mm
      | Surface Area = 2*pi*r*h
      | Density (Stainless Steel 316) = 0.00798 g/mm^3
      | Density (Air) = 1.293e-6 g/mm^3
      | Volume (Stainless Steel 316) = pi*(R^2 - r^2)*h
      | Volume (air) = pi*r^2*h
      | Mass = Volume * Density
  note: Conduction:
      | Thermal Conductivity (Stainless Steel 316) = 16.3 W/K-m
  note: Convection:
      | Heat Transfer Coefficienct = 5 W/K-m^2
  Conductive Heat Transfer Metal : fl_lib/Thermal/Thermal Elements/Conductive Heat Transfer  thermal_type=foundation.enum.ConstantVariableTabulated.Constant  wall_geometry=foundation.enum.ConductionWallGeometry.Planar  area=1507.964 mm^2  thickness=3.1 mm  d_in=0.05 m  d_out=0.1 m  L=1 m  th_cond_min=10 W/(K*m)  th_cond=16.3 W/(K*m)  th_cond_TLU=[413, 401, 392, 383, 371, 357, 342] W/(K*m)  temp_TLU=[200, 273, 400, 600, 800, 1000, 1200] K  T_specify=on  T_priority=None  T=30 degC  T_nominal_specify=off  T_nominal_unit=K  T_nominal_value=1  Q_specify=off  Q_priority=None  Q=0 W  Q_nominal_specify=off  Q_nominal_unit=W  Q_nominal_value=1
  Convective Heat Transfer Metal - Gas - X : fl_lib/Thermal/Thermal Elements/Convective Heat Transfer  thermal_type=foundation.enum.constant_variable.constant  area=1507.964 mm^2  heat_tr_coeff=5 W/(K*m^2)  min_heat_tr_coeff=1e-3 W/(K*m^2)  T_specify=on  T_priority=None  T=30 degC  T_nominal_specify=off  T_nominal_unit=K  T_nominal_value=1  Q_specify=off  Q_priority=None  Q=0 W  Q_nominal_specify=off  Q_nominal_unit=W  Q_nominal_value=1
  Convective Heat Transfer Metal - Gas - Y : fl_lib/Thermal/Thermal Elements/Convective Heat Transfer  thermal_type=foundation.enum.constant_variable.constant  area=1507.964 mm^2  heat_tr_coeff=5 W/(K*m^2)  min_heat_tr_coeff=1e-3 W/(K*m^2)  T_specify=on  T_priority=None  T=30 degC  T_nominal_specify=off  T_nominal_unit=K  T_nominal_value=1  Q_specify=off  Q_priority=None  Q=0 W  Q_nominal_specify=off  Q_nominal_unit=W  Q_nominal_value=1
  Sensor : Subsystem
  Thermal Mass Gas : fl_lib/Thermal/Thermal Elements/Thermal Mass  mass_type=foundation.enum.constant_variable.constant  mass=0.0023 g  sp_heat=715 J/(K*kg)  mass_min=1e-6 kg  num_ports=foundation.enum.numPorts2.one  m_specify=off  m_priority=High  m=1 kg  m_nominal_specify=off  m_nominal_unit=kg  m_nominal_value=1  T_specify=on  T_priority=High  T=30 degC  T_nominal_specify=off  T_nominal_unit=K  T_nominal_value=1  Q_specify=off  Q_priority=None  Q=0 W  Q_nominal_specify=off  Q_nominal_unit=W  Q_nominal_value=1
  Thermal Mass Metal : fl_lib/Thermal/Thermal Elements/Thermal Mass  mass_type=foundation.enum.constant_variable.constant  mass=61.3962 g  sp_heat=468 J/(K*kg)  mass_min=1e-6 kg  num_ports=foundation.enum.numPorts2.one  m_specify=off  m_priority=High  m=1 kg  m_nominal_specify=off  m_nominal_unit=kg  m_nominal_value=1  T_specify=on  T_priority=High  T=30 degC  T_nominal_specify=off  T_nominal_unit=K  T_nominal_value=1  Q_specify=off  Q_priority=None  Q=0 W  Q_nominal_specify=off  Q_nominal_unit=W  Q_nominal_value=1
  A : PMIOPort  Side=Left
  B : PMIOPort  Port=2  Side=Right
  H : PMIOPort  Port=3  Side=Right
  connections:
  H/RConn1 -- Conductive Heat Transfer Metal/LConn1 -- Thermal Mass Metal/LConn1
  Convective Heat Transfer Metal - Gas - Y/RConn1 -- B/RConn1 -- Convective Heat Transfer Metal - Gas - X/RConn1 -- Thermal Mass Gas/LConn1
  Convective Heat Transfer Metal - Gas - Y/LConn1 -- Conductive Heat Transfer Metal/RConn1 -- Sensor/LConn1
  Convective Heat Transfer Metal - Gas - X/LConn1 -- A/RConn1

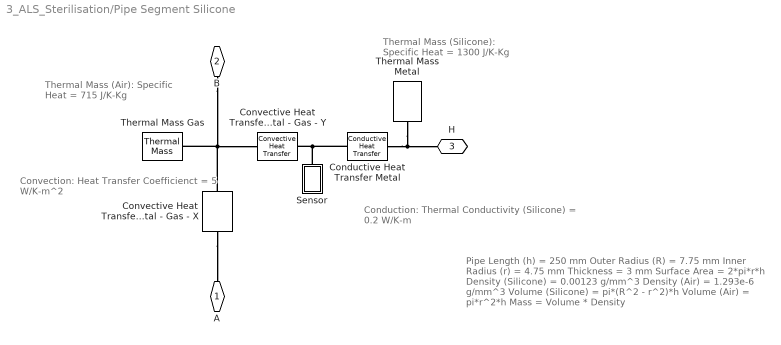
== system 3_ALS_Sterilisation/Pipe Segment Silicone ==
  note: Thermal Mass (Silicone):
      | Specific Heat = 1300 J/K-Kg
  note: Thermal Mass  (Air):
      | Specific Heat = 715 J/K-Kg
  note: Pipe Length (h) = 250 mm
      | Outer Radius (R) = 7.75 mm
      | Inner Radius (r) = 4.75 mm
      | Thickness = 3 mm
      | Surface Area = 2*pi*r*h
      | Density (Silicone) = 0.00123 g/mm^3
      | Density (Air) = 1.293e-6 g/mm^3
      | Volume (Silicone) = pi*(R^2 - r^2)*h
      | Volume (Air) = pi*r^2*h
      | Mass = Volume * Density
  note: Conduction:
      | Thermal Conductivity (Silicone) = 0.2 W/K-m
  note: Convection:
      | Heat Transfer Coefficienct = 5 W/K-m^2
  Conductive Heat Transfer Metal : fl_lib/Thermal/Thermal Elements/Conductive Heat Transfer  thermal_type=foundation.enum.ConstantVariableTabulated.Constant  wall_geometry=foundation.enum.ConductionWallGeometry.Planar  area=7461.282 mm^2  thickness=3 mm  d_in=0.05 m  d_out=0.1 m  L=1 m  th_cond_min=10 W/(K*m)  th_cond=0.2 W/(K*m)  th_cond_TLU=[413, 401, 392, 383, 371, 357, 342] W/(K*m)  temp_TLU=[200, 273, 400, 600, 800, 1000, 1200] K  T_specify=on  T_priority=None  T=20 degC  T_nominal_specify=off  T_nominal_unit=K  T_nominal_value=1  Q_specify=off  Q_priority=None  Q=0 W  Q_nominal_specify=off  Q_nominal_unit=W  Q_nominal_value=1
  Convective Heat Transfer Metal - Gas - X : fl_lib/Thermal/Thermal Elements/Convective Heat Transfer  thermal_type=foundation.enum.constant_variable.constant  area=7461.282 mm^2  heat_tr_coeff=5 W/(K*m^2)  min_heat_tr_coeff=1e-3 W/(K*m^2)  T_specify=on  T_priority=None  T=20 degC  T_nominal_specify=off  T_nominal_unit=K  T_nominal_value=1  Q_specify=off  Q_priority=None  Q=0 W  Q_nominal_specify=off  Q_nominal_unit=W  Q_nominal_value=1
  Convective Heat Transfer Metal - Gas - Y : fl_lib/Thermal/Thermal Elements/Convective Heat Transfer  thermal_type=foundation.enum.constant_variable.constant  area=7461.282 mm^2  heat_tr_coeff=5 W/(K*m^2)  min_heat_tr_coeff=1e-3 W/(K*m^2)  T_specify=on  T_priority=None  T=20 degC  T_nominal_specify=off  T_nominal_unit=K  T_nominal_value=1  Q_specify=off  Q_priority=None  Q=0 W  Q_nominal_specify=off  Q_nominal_unit=W  Q_nominal_value=1
  Sensor : Subsystem
  Thermal Mass Gas : fl_lib/Thermal/Thermal Elements/Thermal Mass  mass_type=foundation.enum.constant_variable.constant  mass=0.0229 g  sp_heat=715 J/(K*kg)  mass_min=1e-6 kg  num_ports=foundation.enum.numPorts2.one  m_specify=off  m_priority=High  m=1 kg  m_nominal_specify=off  m_nominal_unit=kg  m_nominal_value=1  T_specify=on  T_priority=High  T=20 degC  T_nominal_specify=off  T_nominal_unit=K  T_nominal_value=1  Q_specify=off  Q_priority=None  Q=0 W  Q_nominal_specify=off  Q_nominal_unit=W  Q_nominal_value=1
  Thermal Mass Metal : fl_lib/Thermal/Thermal Elements/Thermal Mass  mass_type=foundation.enum.constant_variable.constant  mass=36.2265 g  sp_heat=1300 J/(K*kg)  mass_min=1e-6 kg  num_ports=foundation.enum.numPorts2.one  m_specify=off  m_priority=High  m=1 kg  m_nominal_specify=off  m_nominal_unit=kg  m_nominal_value=1  T_specify=on  T_priority=High  T=20 degC  T_nominal_specify=off  T_nominal_unit=K  T_nominal_value=1  Q_specify=off  Q_priority=None  Q=0 W  Q_nominal_specify=off  Q_nominal_unit=W  Q_nominal_value=1
  A : PMIOPort  Side=Left
  B : PMIOPort  Port=2  Side=Right
  H : PMIOPort  Port=3  Side=Right
  connections:
  Thermal Mass Metal/LConn1 -- H/RConn1 -- Conductive Heat Transfer Metal/LConn1
  Convective Heat Transfer Metal - Gas - X/RConn1 -- Thermal Mass Gas/LConn1 -- Convective Heat Transfer Metal - Gas - Y/RConn1 -- B/RConn1
  Sensor/LConn1 -- Convective Heat Transfer Metal - Gas - Y/LConn1 -- Conductive Heat Transfer Metal/RConn1
  Convective Heat Transfer Metal - Gas - X/LConn1 -- A/RConn1

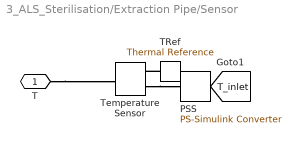
== system 3_ALS_Sterilisation/Extraction Pipe/Sensor ==
  PSS : nesl_utility/PS-Simulink Converter  PhysicalDomain=network_engine_domain  SubClassName=ps_output  LeftPortType=input  RightPortType=output  PseudoPeriodic=off  Frequencies=[]  VectorFormat=1-D array  Unit=1  AffineConversion=off
  TRef : fl_lib/Thermal/Thermal Elements/Thermal Reference
  Temperature Sensor : fl_lib/Thermal/Thermal Sensors/Temperature Sensor  temperature_measure=foundation.enum.MeasurementReference.difference
  T : PMIOPort  Side=Left
  tag scope: T_inlet=global
  wires:
  PSS/1 -> [T_inlet]
  connections:
  T/RConn1 -- Temperature Sensor/LConn1
  TRef/LConn1 -- Temperature Sensor/RConn1
  Temperature Sensor/RConn2 -- PSS/LConn1

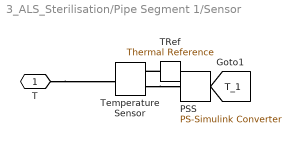
== system 3_ALS_Sterilisation/Pipe Segment 1/Sensor ==
  PSS : nesl_utility/PS-Simulink Converter  PhysicalDomain=network_engine_domain  SubClassName=ps_output  LeftPortType=input  RightPortType=output  PseudoPeriodic=off  Frequencies=[]  VectorFormat=1-D array  Unit=1  AffineConversion=off
  TRef : fl_lib/Thermal/Thermal Elements/Thermal Reference
  Temperature Sensor : fl_lib/Thermal/Thermal Sensors/Temperature Sensor  temperature_measure=foundation.enum.MeasurementReference.difference
  T : PMIOPort  Side=Left
  tag scope: T_1=global
  wires:
  PSS/1 -> [T_1]
  connections:
  T/RConn1 -- Temperature Sensor/LConn1
  TRef/LConn1 -- Temperature Sensor/RConn1
  Temperature Sensor/RConn2 -- PSS/LConn1

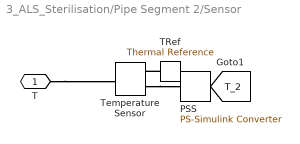
== system 3_ALS_Sterilisation/Pipe Segment 2/Sensor ==
  PSS : nesl_utility/PS-Simulink Converter  PhysicalDomain=network_engine_domain  SubClassName=ps_output  LeftPortType=input  RightPortType=output  PseudoPeriodic=off  Frequencies=[]  VectorFormat=1-D array  Unit=1  AffineConversion=off
  TRef : fl_lib/Thermal/Thermal Elements/Thermal Reference
  Temperature Sensor : fl_lib/Thermal/Thermal Sensors/Temperature Sensor  temperature_measure=foundation.enum.MeasurementReference.difference
  T : PMIOPort  Side=Left
  tag scope: T_2=global
  wires:
  PSS/1 -> [T_2]
  connections:
  T/RConn1 -- Temperature Sensor/LConn1
  TRef/LConn1 -- Temperature Sensor/RConn1
  Temperature Sensor/RConn2 -- PSS/LConn1

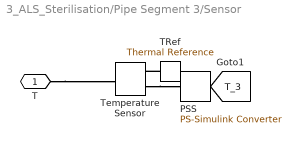
== system 3_ALS_Sterilisation/Pipe Segment 3/Sensor ==
  PSS : nesl_utility/PS-Simulink Converter  PhysicalDomain=network_engine_domain  SubClassName=ps_output  LeftPortType=input  RightPortType=output  PseudoPeriodic=off  Frequencies=[]  VectorFormat=1-D array  Unit=1  AffineConversion=off
  TRef : fl_lib/Thermal/Thermal Elements/Thermal Reference
  Temperature Sensor : fl_lib/Thermal/Thermal Sensors/Temperature Sensor  temperature_measure=foundation.enum.MeasurementReference.difference
  T : PMIOPort  Side=Left
  tag scope: T_3=global
  wires:
  PSS/1 -> [T_3]
  connections:
  T/RConn1 -- Temperature Sensor/LConn1
  TRef/LConn1 -- Temperature Sensor/RConn1
  Temperature Sensor/RConn2 -- PSS/LConn1

== system 3_ALS_Sterilisation/Pipe Segment 4/Sensor ==
  PSS : nesl_utility/PS-Simulink Converter  PhysicalDomain=network_engine_domain  SubClassName=ps_output  LeftPortType=input  RightPortType=output  PseudoPeriodic=off  Frequencies=[]  VectorFormat=1-D array  Unit=1  AffineConversion=off
  TRef : fl_lib/Thermal/Thermal Elements/Thermal Reference
  Temperature Sensor : fl_lib/Thermal/Thermal Sensors/Temperature Sensor  temperature_measure=foundation.enum.MeasurementReference.difference
  T : PMIOPort  Side=Left
  tag scope: T_4=global
  wires:
  PSS/1 -> [T_4]
  connections:
  T/RConn1 -- Temperature Sensor/LConn1
  TRef/LConn1 -- Temperature Sensor/RConn1
  Temperature Sensor/RConn2 -- PSS/LConn1

== system 3_ALS_Sterilisation/Pipe Segment 5/Sensor ==
  PSS : nesl_utility/PS-Simulink Converter  PhysicalDomain=network_engine_domain  SubClassName=ps_output  LeftPortType=input  RightPortType=output  PseudoPeriodic=off  Frequencies=[]  VectorFormat=1-D array  Unit=1  AffineConversion=off
  TRef : fl_lib/Thermal/Thermal Elements/Thermal Reference
  Temperature Sensor : fl_lib/Thermal/Thermal Sensors/Temperature Sensor  temperature_measure=foundation.enum.MeasurementReference.difference
  T : PMIOPort  Side=Left
  tag scope: T_5=global
  wires:
  PSS/1 -> [T_5]
  connections:
  T/RConn1 -- Temperature Sensor/LConn1
  TRef/LConn1 -- Temperature Sensor/RConn1
  Temperature Sensor/RConn2 -- PSS/LConn1

== system 3_ALS_Sterilisation/Pipe Segment Silicone/Sensor ==
  PSS : nesl_utility/PS-Simulink Converter  PhysicalDomain=network_engine_domain  SubClassName=ps_output  LeftPortType=input  RightPortType=output  PseudoPeriodic=off  Frequencies=[]  VectorFormat=1-D array  Unit=1  AffineConversion=off
  TRef : fl_lib/Thermal/Thermal Elements/Thermal Reference
  Temperature Sensor : fl_lib/Thermal/Thermal Sensors/Temperature Sensor  temperature_measure=foundation.enum.MeasurementReference.difference
  T : PMIOPort  Side=Left
  tag scope: T_2=global
  wires:
  PSS/1 -> [T_2]
  connections:
  T/RConn1 -- Temperature Sensor/LConn1
  TRef/LConn1 -- Temperature Sensor/RConn1
  Temperature Sensor/RConn2 -- PSS/LConn1
